simulink model "Subsystem"  (R2020b)
settings: Solver=FixedStepAuto  StartTime=0.0  StopTime=10.0  FixedStep=5  RelTol=1e-3
settings Model: Creator=Pulkit Khandelwal  LastModifiedBy=Pulkit Khandelwal
settings DataIOCC: SaveOutput=off  SaveTime=off

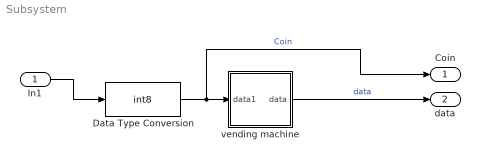
== system Subsystem ==
  In1 : Inport  OutDataTypeStr=double  PortDimensions=1  SampleTime=[5,0]
  Data Type Conversion : DataTypeConversion  OutDataTypeStr=int8  RndMeth=Nearest  SaturateOnIntegerOverflow=on
  vending machine : Stateflow chart  TreatAsAtomicUnit=on
  Coin : Outport  OutDataTypeStr=int8  PortDimensions=1  SampleTime=[5,0]
  data : Outport  Port=2  OutDataTypeStr=double  PortDimensions=1  SampleTime=[5,0]
  wires:
  Data Type Conversion/1 -> vending machine/1(data1), Coin/1  "Coin"
  In1/1 -> Data Type Conversion/1
  vending machine/1(data) -> data/1  "data"

== stateflow chart Subsystem/vending machine ==
  settings: stateMachineType=MEALY_MACHINE
  state Got_0
  state Got_Nickel
  state Got_Dime
  (default) -> Got_0
  Got_0 -> Got_Nickel [order 1] : [data1==1]{data=0}
  Got_Nickel -> Got_0 [order 1] : [data1==2]{data=1}
  Got_Dime -> Got_0 [order 2] : [data1==1]{data=1}
  Got_0 -> Got_Dime [order 2] : [data1==2]{data=0}
  Got_Nickel -> Got_Dime [order 2] : [data1==1]{data=0}
  Got_Dime -> Got_Nickel [order 1] : [data1==2]{data=1}
  data: data output; data1 input
